simulink model "EnabledandTriggerSubsystem"  (R2015b)
settings: Solver=FixedStepAuto  StartTime=0.0  StopTime=10.0  FixedStep=0.25  RelTol=1e-3
PreLoadFcn:
  | loadvar
StartFcn:
  | open_scope
settings Model: Creator=LUBO  LastModifiedBy=LUBO

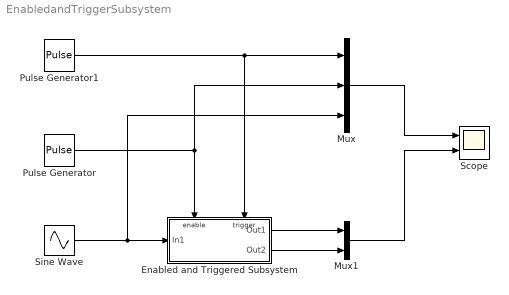
== system EnabledandTriggerSubsystem ==
  Enabled and Triggered Subsystem : Subsystem  TreatAsAtomicUnit=on
      settings: DeleteFcn=msgbox('This block is being deleted!')  OpenFcn=loadvar
  Mux : Mux  Inputs=3
  Mux1 : Mux  Inputs=2
  Pulse Generator : DiscretePulseGenerator  Period=20  PulseWidth=10  SampleTime=0.25
  Pulse Generator1 : DiscretePulseGenerator  SampleTime=0.25
  Scope : Scope  NumInputPorts=2
  Sine Wave : Sin  SineType=Sample based  Samples=20  SampleTime=0.25
  wires:
  Pulse Generator1/1 -> Enabled and Triggered Subsystem/Trigger, Mux/1
  Pulse Generator/1 -> Enabled and Triggered Subsystem/Enable, Mux/2
  Sine Wave/1 -> Mux/3, Enabled and Triggered Subsystem/1(In1)
  Enabled and Triggered Subsystem/1(Out1) -> Mux1/1
  Enabled and Triggered Subsystem/2(Out2) -> Mux1/2
  Mux/1 -> Scope/1
  Mux1/1 -> Scope/2

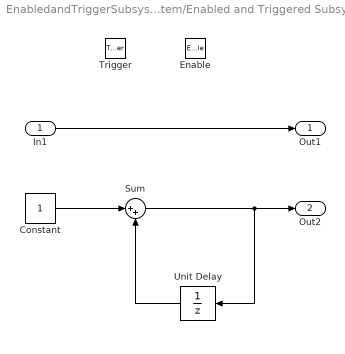
== system EnabledandTriggerSubsystem/Enabled and Triggered Subsystem ==
  In1 : Inport
  Enable : EnablePort
  Trigger : TriggerPort
  Constant : Constant
  Sum : Sum  Inputs=|++
  Unit Delay : UnitDelay  SampleTime=-1
  Out1 : Outport  InitialOutput=0
  Out2 : Outport  Port=2  InitialOutput=0
  wires:
  In1/1 -> Out1/1
  Constant/1 -> Sum/1
  Sum/1 -> Unit Delay/1, Out2/1
  Unit Delay/1 -> Sum/2
